simulink model "s1o"  (Simulink 2.00)
settings: Solver=ode113  StartTime=0.0  StopTime=tstop  MaxStep=1e-2  RelTol=1e-5  AbsTol=1e-6
values from neighbouring files (symbols this model uses):
  H = J*wbm*wbm/(2*Sb)    (= 3.33396824273)    [P20HP.M]
  P = 4    [P20HP.M]
  Psidso = 0    [M1C.M]    (also in M1O.M; M3.M)
  Psipdro = 0    [M1C.M]    (also in M1O.M; M3.M)
  Psipqro = 0    [M1C.M]    (also in M1O.M; M3.M)
  Psiqso = 0    [M1C.M]    (also in M1O.M; M3.M)
  rpr = 0.0764    [P20HP.M]
  rs = 0.1062    [P20HP.M]
  time_tmech = [0 4]    [M1C.M]    (also in M1O.M = [0 0.75 0.75 1.0 1.0 1.25 1.25 1.5 1.5 2]; M3.M = [0 tstop])
  tmech_tmech = [0 0]    [M1C.M]    (also in M1O.M = [0 0 -Trated -Trated -Trated/2 -Trated/2 -Trated -Trated 0 0; M3.M)
  Vb = Vm    [P20HP.M]
  wb = 2*pi*frated    (= 376.991118431)    [P20HP.M]
  we = w(n)    [M1C.M]    (also in M1O.M; M3.M = wb; P20HP.M = 376.991118431)
  xls = (we/wb)*xls    [M1C.M]    (also in M1O.M; M3.M; P20HP.M = 0.2145)
  xM = 1/(1/xm + 1/xls + 1/xplr)    [M1C.M]    (also in M1O.M; M3.M; P20HP.M = 0.105313916498)
  xplr = (we/wb)*xplr    [M1C.M]    (also in M1O.M; M3.M; P20HP.M = 0.2145)
  Zb = Vrated*Vrated/Sb    (= 3.24396782842)    [P20HP.M]
settings Model: SaveTime=off  SaveOutput=off  ConsistencyChecking=off

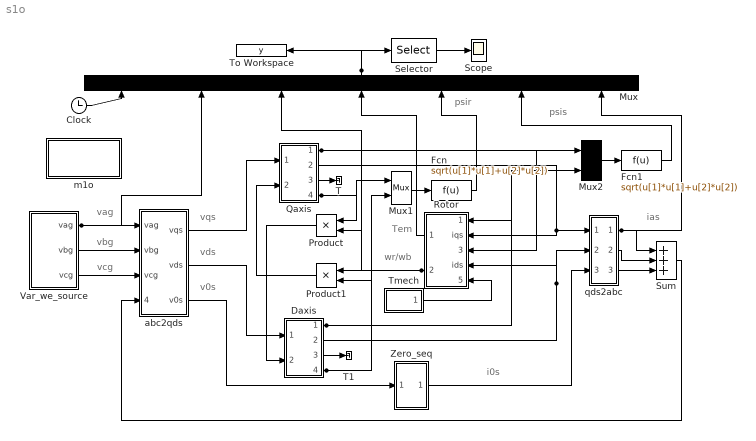
== system s1o ==
  note: wr/wb
  note: Tem
  note: vag
  note: vqs
  note: vds
  note: v0s
  note: vcg
  note: vbg
  note: i0s
  note: ias
  note: psir
  note: psis
  Clock : Clock
      settings: DeleteFcn=simclock BlockIsBeingDestroyed  PostSaveFcn=simclock Save
  Daxis : Subsystem
  Fcn : Fcn  Expr=sqrt(u[1]*u[1]+u[2]*u[2])
  Fcn1 : Fcn  Expr=sqrt(u[1]*u[1]+u[2]*u[2])
  m1o : Subsystem
      settings: OpenFcn=m1o
      mask Type: Masked block of m1o.m
      mask Help: Uses m1o.m to initialize and plot
      mask Display: disp('Initialize\nand plot')
  Mux : Mux  Orientation=up  Inputs=7
  Mux1 : Mux  Inputs=2
  Mux2 : Mux  Inputs=2
  Product : Product  Orientation=left  Inputs=2
  Product1 : Product  Orientation=left  Inputs=2
  Qaxis : Subsystem
  Rotor : Subsystem  Orientation=left
  Scope : Scope
      settings: TickLabels=on  TimeRange=2  YMin=-200  YMax=200  SaveToWorkspace=off  SaveName=ScopeData  LimitMaxRows=off
  Selector : Selector  Elements=[2 3 4 5 6 7]  InputPortWidth=7
  Sum : Sum  Inputs=+++
  T : Terminator
  T1 : Terminator
  Tmech : Subsystem  mask(Repeating table){rep_seq_t=time_tmech, rep_seq_y=tmech_tmech}
      mask prompts: rep_seq_t "Time values:"; rep_seq_y "Output values:"
      mask help: Repeating table.
      mask init:
      | period = max(rep_seq_t);
      mask Help: Repeats cycle given in table. Time values should be monotonically increasing.
      mask Display: plot([rep_seq_t,rep_seq_t+period,rep_seq_t+2*period,rep_seq_t(1)+3*period],[rep_seq_y,rep_seq_y,rep_seq_y,rep_seq_y(1)])
  To Workspace : ToWorkspace  VariableName=y  SampleTime=0
      settings: Buffer=40000
  Var_we_source : Subsystem
  Zero_seq : Subsystem
  abc2qds : Subsystem
  qds2abc : Subsystem
  wires:
  Daxis/2(out_ids) -> qds2abc/2(ids), Rotor/4(ids)
  Product1/1 -> Qaxis/2(in_(wr/wb)*psidr')
  abc2qds/2(vds) -> Daxis/1(in_vds)
  abc2qds/1(vqs) -> Qaxis/1(in_vqs)
  Qaxis/2(out_iqs) -> qds2abc/1(iqs), Rotor/2(iqs)
  Product/1 -> Daxis/2(in_(wr/wb)*psiqr')
  Rotor/2(wr/wb) -> Product/2, Product1/1, Mux/3
  Tmech/1(out_1) -> Rotor/5(Tmech)
  Clock/1 -> Mux/1
  Var_we_source/2(vbg) -> abc2qds/2(vbg)
  Var_we_source/3(vcg) -> abc2qds/3(vcg)
  Zero_seq/1(i0s) -> qds2abc/3(i0s)
  qds2abc/2(ibs) -> Sum/2
  qds2abc/3(ics) -> Sum/3
  abc2qds/3(v0s) -> Zero_seq/1(v0s)
  Sum/1 -> abc2qds/4(ias+ibs+ics)
  Mux1/1 -> Fcn/1
  Mux2/1 -> Fcn1/1
  Qaxis/1(out_psiqs) -> Rotor/3(psiqs), Mux2/1
  Daxis/1(out_psids) -> Rotor/1(psids), Mux2/2
  Var_we_source/1(vag) -> abc2qds/1(vag), Mux/2
  Rotor/1(Tem_out) -> Mux/4
  Fcn/1 -> Mux/5
  Fcn1/1 -> Mux/6
  qds2abc/1(ias) -> Sum/1, Mux/7
  Qaxis/4(out_psiqr') -> Product/1, Mux1/1
  Daxis/4(out_psidr') -> Product1/2, Mux1/2
  Qaxis/3(out_iqr') -> T/1
  Daxis/3(out_idr') -> T1/1
  Selector/1 -> Scope/1
  Mux/1 -> To Workspace/1, Selector/1

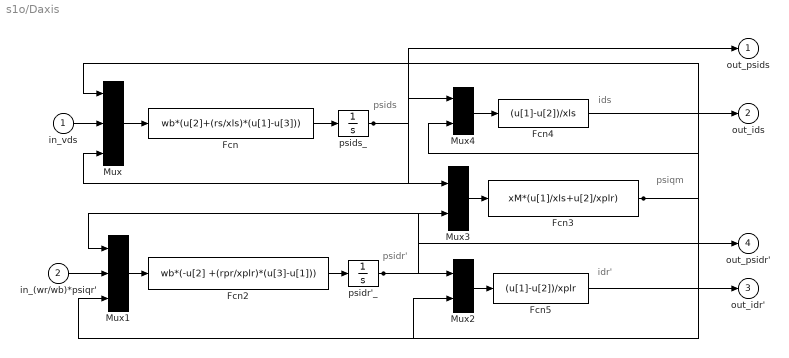
== system s1o/Daxis ==
  note: ids
  note: psids
  note: psiqm
  note: idr'
  note: psidr'
  in_vds : Inport  Port=1  PortWidth=-1  SampleTime=-1
  in_(wr/wb)*psiqr' : Inport  Port=2  PortWidth=-1  SampleTime=-1
  Fcn : Fcn  Expr=wb*(u[2]+(rs/xls)*(u[1]-u[3]))
  Fcn2 : Fcn  Expr=wb*(-u[2] +(rpr/xplr)*(u[3]-u[1]))
  Fcn3 : Fcn  Expr=xM*(u[1]/xls+u[2]/xplr)
  Fcn4 : Fcn  Expr=(u[1]-u[2])/xls
  Fcn5 : Fcn  Expr=(u[1]-u[2])/xplr
  Mux : Mux  Inputs=3
  Mux1 : Mux  Inputs=3
  Mux2 : Mux  Inputs=2
  Mux3 : Mux  Inputs=2
  Mux4 : Mux  Inputs=2
  psidr'_ : Integrator  ExternalReset=none  InitialConditionSource=internal  InitialCondition=Psipdro  LimitOutput=off  UpperSaturationLimit=inf  LowerSaturationLimit=-inf  ShowSaturationPort=off  ShowStatePort=off  AbsoluteTolerance=auto
  psids_ : Integrator  ExternalReset=none  InitialConditionSource=internal  InitialCondition=Psidso  LimitOutput=off  UpperSaturationLimit=inf  LowerSaturationLimit=-inf  ShowSaturationPort=off  ShowStatePort=off  AbsoluteTolerance=auto
  out_psids : Outport  Port=1  InitialOutput=0
  out_ids : Outport  Port=2  InitialOutput=0
  out_idr' : Outport  Port=3  InitialOutput=0
  out_psidr' : Outport  Port=4  InitialOutput=0
  wires:
  Mux2/1 -> Fcn5/1
  psidr'_/1 -> Mux2/1, Mux3/2, Mux1/1, out_psidr'/1
  Mux1/1 -> Fcn2/1
  Fcn3/1 -> Mux2/2, Mux/1, Mux1/3, Mux4/2
  psids_/1 -> Mux/3, Mux4/1, Mux3/1, out_psids/1
  Mux4/1 -> Fcn4/1
  Mux3/1 -> Fcn3/1
  Fcn2/1 -> psidr'_/1
  Fcn/1 -> psids_/1
  Mux/1 -> Fcn/1
  Fcn4/1 -> out_ids/1
  in_vds/1 -> Mux/2
  in_(wr/wb)*psiqr'/1 -> Mux1/2
  Fcn5/1 -> out_idr'/1

== system s1o/m1o ==
  note: masked block of m1o.m
      | to initilialize s1o.m
      | and to plot the results.

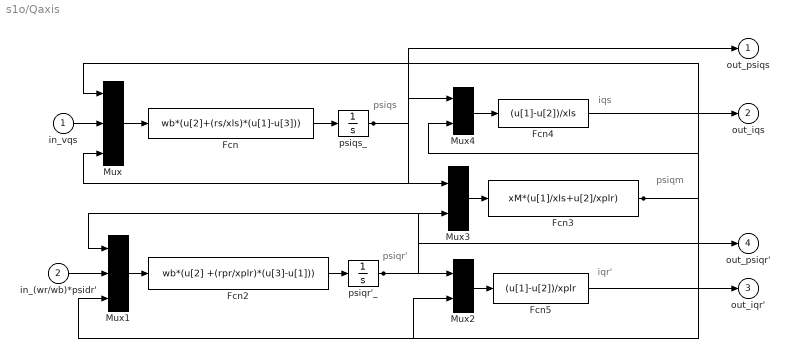
== system s1o/Qaxis ==
  note: iqs
  note: psiqs
  note: psiqm
  note: iqr'
  note: psiqr'
  in_vqs : Inport  Port=1  PortWidth=-1  SampleTime=-1
  in_(wr/wb)*psidr' : Inport  Port=2  PortWidth=-1  SampleTime=-1
  Fcn : Fcn  Expr=wb*(u[2]+(rs/xls)*(u[1]-u[3]))
  Fcn2 : Fcn  Expr=wb*(u[2] +(rpr/xplr)*(u[3]-u[1]))
  Fcn3 : Fcn  Expr=xM*(u[1]/xls+u[2]/xplr)
  Fcn4 : Fcn  Expr=(u[1]-u[2])/xls
  Fcn5 : Fcn  Expr=(u[1]-u[2])/xplr
  Mux : Mux  Inputs=3
  Mux1 : Mux  Inputs=3
  Mux2 : Mux  Inputs=2
  Mux3 : Mux  Inputs=2
  Mux4 : Mux  Inputs=2
  psiqr'_ : Integrator  ExternalReset=none  InitialConditionSource=internal  InitialCondition=Psipqro  LimitOutput=off  UpperSaturationLimit=inf  LowerSaturationLimit=-inf  ShowSaturationPort=off  ShowStatePort=off  AbsoluteTolerance=auto
  psiqs_ : Integrator  ExternalReset=none  InitialConditionSource=internal  InitialCondition=Psiqso  LimitOutput=off  UpperSaturationLimit=inf  LowerSaturationLimit=-inf  ShowSaturationPort=off  ShowStatePort=off  AbsoluteTolerance=auto
  out_psiqs : Outport  Port=1  InitialOutput=0
  out_iqs : Outport  Port=2  InitialOutput=0
  out_iqr' : Outport  Port=3  InitialOutput=0
  out_psiqr' : Outport  Port=4  InitialOutput=0
  wires:
  Mux2/1 -> Fcn5/1
  psiqr'_/1 -> Mux2/1, Mux3/2, Mux1/1, out_psiqr'/1
  Mux1/1 -> Fcn2/1
  Fcn3/1 -> Mux2/2, Mux/1, Mux1/3, Mux4/2
  psiqs_/1 -> Mux/3, Mux4/1, Mux3/1, out_psiqs/1
  Mux4/1 -> Fcn4/1
  Mux3/1 -> Fcn3/1
  Fcn2/1 -> psiqr'_/1
  Fcn/1 -> psiqs_/1
  Mux/1 -> Fcn/1
  Fcn4/1 -> out_iqs/1
  in_vqs/1 -> Mux/2
  in_(wr/wb)*psidr'/1 -> Mux1/2
  Fcn5/1 -> out_iqr'/1

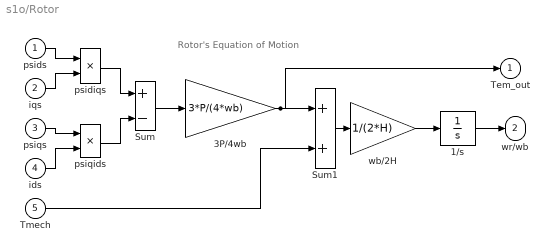
== system s1o/Rotor ==
  note: Rotor's Equation of Motion
  psids : Inport  Port=1  PortWidth=-1  SampleTime=-1
  iqs : Inport  Port=2  PortWidth=-1  SampleTime=-1
  psiqs : Inport  Port=3  PortWidth=-1  SampleTime=-1
  ids : Inport  Port=4  PortWidth=-1  SampleTime=-1
  Tmech : Inport  Port=5  PortWidth=-1  SampleTime=-1
  1/s : Integrator  ExternalReset=none  InitialConditionSource=internal  InitialCondition=0  LimitOutput=off  UpperSaturationLimit=inf  LowerSaturationLimit=-inf  ShowSaturationPort=off  ShowStatePort=off  AbsoluteTolerance=auto
  3P/4wb : Gain  Gain=3*P/(4*wb)
  Sum : Sum  Inputs=+-
  Sum1 : Sum  Inputs=++
  psidiqs : Product  Inputs=2
  psiqids : Product  Inputs=2
  wb/2H : Gain  Gain=1/(2*H)
  Tem_out : Outport  Port=1  InitialOutput=0
  wr/wb : Outport  Port=2  InitialOutput=0
  wires:
  Sum/1 -> 3P/4wb/1
  psiqs/1 -> psiqids/1
  iqs/1 -> psidiqs/2
  psids/1 -> psidiqs/1
  psidiqs/1 -> Sum/1
  psiqids/1 -> Sum/2
  1/s/1 -> wr/wb/1
  Tmech/1 -> Sum1/2
  ids/1 -> psiqids/2
  Sum1/1 -> wb/2H/1
  wb/2H/1 -> 1/s/1
  3P/4wb/1 -> Sum1/1, Tem_out/1

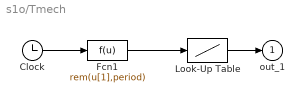
== system s1o/Tmech ==
  Clock : Clock
      settings: DeleteFcn=simclock BlockIsBeingDestroyed  PostSaveFcn=simclock Save
  Fcn1 : Fcn  Expr=rem(u[1],period)
  Look-Up Table : Lookup  InputValues=rep_seq_t  OutputValues=rep_seq_y
  out_1 : Outport  Port=1  InitialOutput=0
  wires:
  Look-Up Table/1 -> out_1/1
  Clock/1 -> Fcn1/1
  Fcn1/1 -> Look-Up Table/1

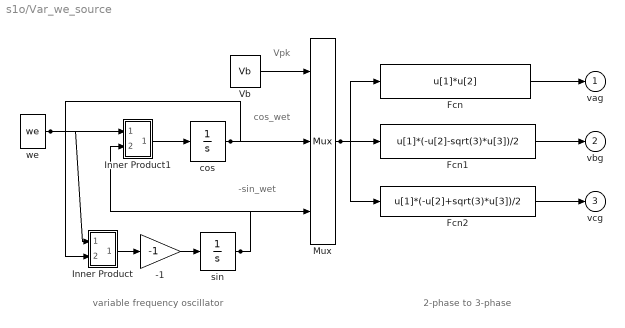
== system s1o/Var_we_source ==
  note: variable frequency oscillator
  note: Vpk
  note: 2-phase to 3-phase
  note: -sin_wet
  note: cos_wet
  -1 : Gain  Gain=-1
  Fcn : Fcn  Expr=u[1]*u[2]
  Fcn1 : Fcn  Expr=u[1]*(-u[2]-sqrt(3)*u[3])/2
  Fcn2 : Fcn  Expr=u[1]*(-u[2]+sqrt(3)*u[3])/2
  Inner Product : Subsystem
      mask Type: Dot Product
      mask Description:
      | Inner (dot) product.
      | y=sum(u1.*u2)
      mask Help: Computes the inner (dot) product of the inputs: sum(u1.*u2).  The inputs are vectors of the same length. Output is a scalar.
      mask Display: disp('.\n')
  Inner Product1 : Subsystem
      mask Type: Dot Product
      mask Description:
      | Inner (dot) product.
      | y=sum(u1.*u2)
      mask Help: Computes the inner (dot) product of the inputs: sum(u1.*u2).  The inputs are vectors of the same length. Output is a scalar.
      mask Display: disp('.\n')
  Mux : Mux  Inputs=3
  Vb : Constant  Value=Vb
  cos : Integrator  ExternalReset=none  InitialConditionSource=internal  InitialCondition=1  LimitOutput=off  UpperSaturationLimit=inf  LowerSaturationLimit=-inf  ShowSaturationPort=off  ShowStatePort=off  AbsoluteTolerance=auto
  sin : Integrator  ExternalReset=none  InitialConditionSource=internal  InitialCondition=0  LimitOutput=off  UpperSaturationLimit=inf  LowerSaturationLimit=-inf  ShowSaturationPort=off  ShowStatePort=off  AbsoluteTolerance=auto
  we : Constant  Value=we
  vag : Outport  Port=1  InitialOutput=0
  vbg : Outport  Port=2  InitialOutput=0
  vcg : Outport  Port=3  InitialOutput=0
  wires:
  we/1 -> Inner Product1/1(in_1), Inner Product/1(in_1)
  -1/1 -> sin/1
  Inner Product/1(out_1) -> -1/1
  Inner Product1/1(out_1) -> cos/1
  cos/1 -> Inner Product/2(in_2), Mux/2
  sin/1 -> Inner Product1/2(in_2), Mux/3
  Fcn/1 -> vag/1
  Fcn1/1 -> vbg/1
  Fcn2/1 -> vcg/1
  Mux/1 -> Fcn/1, Fcn1/1, Fcn2/1
  Vb/1 -> Mux/1

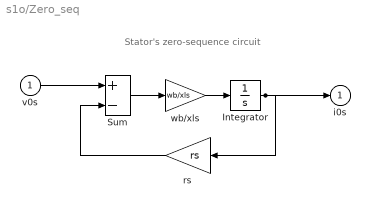
== system s1o/Zero_seq ==
  note: Stator's zero-sequence circuit
  v0s : Inport  Port=1  PortWidth=-1  SampleTime=-1
  Integrator : Integrator  ExternalReset=none  InitialConditionSource=internal  InitialCondition=0  LimitOutput=off  UpperSaturationLimit=inf  LowerSaturationLimit=-inf  ShowSaturationPort=off  ShowStatePort=off  AbsoluteTolerance=auto
  Sum : Sum  Inputs=+-
  rs : Gain  Orientation=left  Gain=rs
  wb/xls : Gain  Gain=wb/xls
  i0s : Outport  Port=1  InitialOutput=0
  wires:
  rs/1 -> Sum/2
  Sum/1 -> wb/xls/1
  wb/xls/1 -> Integrator/1
  v0s/1 -> Sum/1
  Integrator/1 -> rs/1, i0s/1

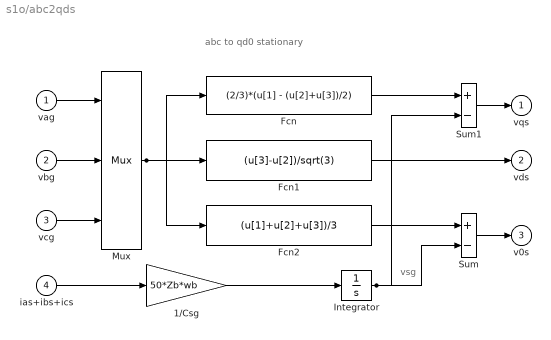
== system s1o/abc2qds ==
  note: abc to qd0 stationary
  note: vsg
  vag : Inport  Port=1  PortWidth=-1  SampleTime=-1
  vbg : Inport  Port=2  PortWidth=-1  SampleTime=-1
  vcg : Inport  Port=3  PortWidth=-1  SampleTime=-1
  ias+ibs+ics : Inport  Port=4  PortWidth=-1  SampleTime=-1
  1/Csg : Gain  Gain=50*Zb*wb
  Fcn : Fcn  Expr=(2/3)*(u[1] - (u[2]+u[3])/2)
  Fcn1 : Fcn  Expr=(u[3]-u[2])/sqrt(3)
  Fcn2 : Fcn  Expr=(u[1]+u[2]+u[3])/3
  Integrator : Integrator  ExternalReset=none  InitialConditionSource=internal  InitialCondition=0  LimitOutput=off  UpperSaturationLimit=inf  LowerSaturationLimit=-inf  ShowSaturationPort=off  ShowStatePort=off  AbsoluteTolerance=auto
  Mux : Mux  Inputs=3
  Sum : Sum  Inputs=+-
  Sum1 : Sum  Inputs=+-
  vqs : Outport  Port=1  InitialOutput=0
  vds : Outport  Port=2  InitialOutput=0
  v0s : Outport  Port=3  InitialOutput=0
  wires:
  ias+ibs+ics/1 -> 1/Csg/1
  vag/1 -> Mux/1
  vbg/1 -> Mux/2
  vcg/1 -> Mux/3
  Mux/1 -> Fcn1/1, Fcn/1, Fcn2/1
  Fcn1/1 -> vds/1
  Sum/1 -> v0s/1
  Fcn2/1 -> Sum/1
  1/Csg/1 -> Integrator/1
  Fcn/1 -> Sum1/1
  Sum1/1 -> vqs/1
  Integrator/1 -> Sum/2, Sum1/2

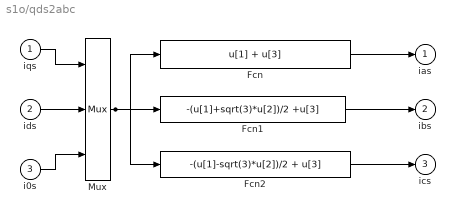
== system s1o/qds2abc ==
  iqs : Inport  Port=1  PortWidth=-1  SampleTime=-1
  ids : Inport  Port=2  PortWidth=-1  SampleTime=-1
  i0s : Inport  Port=3  PortWidth=-1  SampleTime=-1
  Fcn : Fcn  Expr=u[1] + u[3]
  Fcn1 : Fcn  Expr=-(u[1]+sqrt(3)*u[2])/2 +u[3]
  Fcn2 : Fcn  Expr=-(u[1]-sqrt(3)*u[2])/2 + u[3]
  Mux : Mux  Inputs=3
  ias : Outport  Port=1  InitialOutput=0
  ibs : Outport  Port=2  InitialOutput=0
  ics : Outport  Port=3  InitialOutput=0
  wires:
  ids/1 -> Mux/2
  iqs/1 -> Mux/1
  i0s/1 -> Mux/3
  Fcn1/1 -> ibs/1
  Fcn/1 -> ias/1
  Mux/1 -> Fcn1/1, Fcn/1, Fcn2/1
  Fcn2/1 -> ics/1

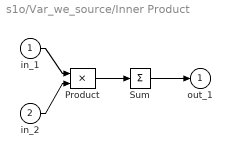
== system s1o/Var_we_source/Inner Product ==
  in_1 : Inport  Port=1  PortWidth=-1  SampleTime=-1
  in_2 : Inport  Port=2  PortWidth=-1  SampleTime=-1
  Product : Product  Inputs=2
  Sum : Sum  Inputs=+
  out_1 : Outport  Port=1  InitialOutput=0
  wires:
  in_2/1 -> Product/2
  in_1/1 -> Product/1
  Product/1 -> Sum/1
  Sum/1 -> out_1/1

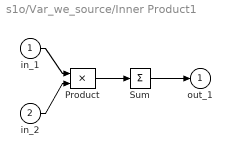
== system s1o/Var_we_source/Inner Product1 ==
  in_1 : Inport  Port=1  PortWidth=-1  SampleTime=-1
  in_2 : Inport  Port=2  PortWidth=-1  SampleTime=-1
  Product : Product  Inputs=2
  Sum : Sum  Inputs=+
  out_1 : Outport  Port=1  InitialOutput=0
  wires:
  in_2/1 -> Product/2
  in_1/1 -> Product/1
  Product/1 -> Sum/1
  Sum/1 -> out_1/1
